simulink model "battery_control"  (R2019a)
settings: Solver=VariableStepAuto  StartTime=0.0  StopTime=10.0  RelTol=1e-3
undefined symbols (not defined in the file or in its folder): Ion, Lithium
libraries: powerlib x6, electricdrivelib x1
settings Model: Creator=nitbh  LastModifiedBy=nitbh

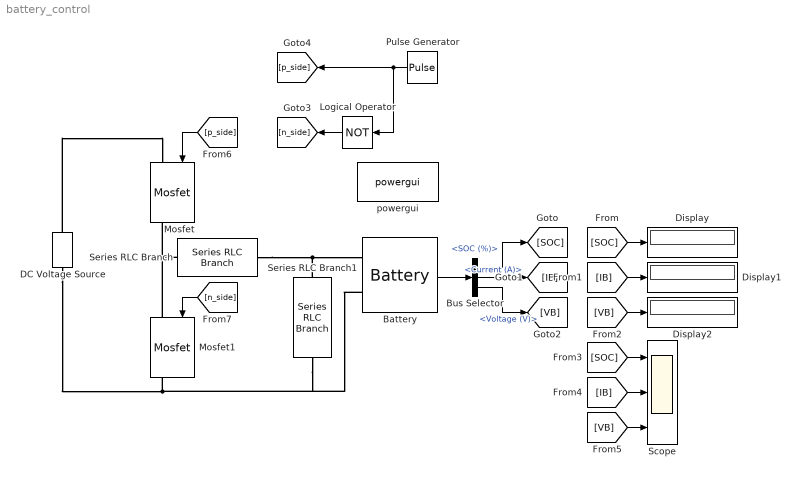
== system battery_control ==
  Battery : electricdrivelib/Extra Sources/Battery  BatType=Lithium-Ion  ShowTempParam=off  ThermalPreset=no  ShowAgeParam=off  NomV=24  NomQ=10  SOC=50  Batt_Tr=30  PresetModel=on  MaxQ=10  MinV=18  FullV=27.9357  Dis_rate=4.3478  R=0.024  Normal_OP=9.0435  expZone="[25.9293     0.491304]"  current=[6.5 13 32.5]  Units=Time  Tci=20  NomT=20  T2=-30  MaxQ2=4.8  FullV2=7.1  Normal_OP2=5.655  expZone2="[6.58           1]"  Rca=0.6  ti=2000  Dp=0  Neq0=0  Tsim=1e6  Ta1=25  Qeol=5.4*0.9  Reol=0.013333*1.2  Char_age=[2.3478, 3]  Dis_age=[2.3478, 10]  N1=1500  N2=10500  N3=1000  N4=1400  Ta2=45  N5=950
      settings: SourceProductName=Simscape Electrical
  Bus Selector : BusSelector  OutputSignals=SOC (%),Current (A),Voltage (V)
  DC Voltage Source : powerlib/Electrical Sources/DC Voltage Source  Amplitude=48  Measurements=None
      settings: SourceProductName=Simscape Electrical
  Display : Display
  Display1 : Display
  Display2 : Display
  Logical Operator : Logic  Operator=NOT  AllPortsSameDT=off  OutDataTypeStr=boolean
  Mosfet : powerlib/Power Electronics/Mosfet  Ron=0.1  Lon=0  Rd=0.01  Vfd=0  IC=0  Rs=1e5  Cs=inf  Measurements=on
      settings: SourceProductName=Simscape Electrical
  Mosfet1 : powerlib/Power Electronics/Mosfet  Ron=0.1  Lon=0  Rd=0.01  Vfd=0  IC=0  Rs=1e5  Cs=inf  Measurements=on
      settings: SourceProductName=Simscape Electrical
  Pulse Generator : DiscretePulseGenerator  PulseType=Time based  Period=1e-4  PulseWidth=50
  Scope : Scope  NumInputPorts=3
  Series RLC Branch : powerlib/Elements/Series RLC Branch  LConnTagsString=__new0  RConnTagsString=__new0  BranchType=RL  Resistance=0.1  Inductance=1e-3  SetiL0=off  InitialCurrent=0  Capacitance=1e-6  Setx0=off  InitialVoltage=0  Measurements=None
      settings: SourceProductName=Simscape Electrical
  Series RLC Branch1 : powerlib/Elements/Series RLC Branch  LConnTagsString=__new0  RConnTagsString=__new0  BranchType=RC  Resistance=0.001  Inductance=1e-3  SetiL0=off  InitialCurrent=0  Capacitance=1000e-6  Setx0=off  InitialVoltage=0  Measurements=None
      settings: SourceProductName=Simscape Electrical
  powergui : powerlib/powergui  Priority=1  SimulationMode=Discrete  SampleTime=5e-6  frequency=60  Iterations=50  frequencyindice=0  Pbase=100e6  ErrMax=1e-4  UnitsV=kV  UnitsW=MW  buscounter=0  FunctionMessages=off  echomessages=off  EnableUseOfTLC=off  CurrentSourceSwitches=off  DisableSnubberDevices=off  DisableRonSwitches=off  DisableVfSwitches=off  DisplayEquations=off  AutomaticDiscreteSolvers=off  SolverType=Tustin/Backward Euler (TBE)  Interpol=off  ExternalGateDelay=off  methode=off  Ts=100  x0status=blocks  SPID=on  SwTol=0  HookPort=off  NonlinearTolerance=0  nMaxIteration=15  ContinueOnMaxIteration=off  RestoreLinks=warning  ResistiveCurrentMeasurement=off  Frange=[0:2:500]  Ylog=off  Xlog=on  ShowGrid=off  save=off  variable=ZData  structure=0  ZoomFFT=off  StartTime=0.0  cycles=1  DisplayStyle=1  fundamental=60  FreqAxis=off  MaxFrequency=1000  frequencyindicesteady=1  RmsSteady=1  display=off
      settings: SourceProductName=Simscape Electrical
  wires:
  Battery/1 -> Bus Selector/1
  Bus Selector/1 -> [SOC]  "<SOC (%)>"
  Bus Selector/2 -> [IB]  "<Current (A)>"
  Bus Selector/3 -> [VB]  "<Voltage (V)>"
  [SOC] -> Display/1
  [VB] -> Display2/1
  [IB] -> Display1/1
  [IB] -> Scope/2
  [VB] -> Scope/3
  [SOC] -> Scope/1
  Pulse Generator/1 -> Logical Operator/1, [p_side]
  Logical Operator/1 -> [n_side]
  [n_side] -> Mosfet1/1
  [p_side] -> Mosfet/1
  connections:
  Mosfet1/LConn1 -- Series RLC Branch/LConn1 -- Mosfet/RConn1
  DC Voltage Source/LConn1 -- Series RLC Branch1/RConn1 -- Battery/LConn2 -- Mosfet1/RConn1
  Series RLC Branch/RConn1 -- Series RLC Branch1/LConn1 -- Battery/LConn1
  DC Voltage Source/RConn1 -- Mosfet/LConn1
